simulink model "Modelo_Diferencial"  (R2019a)
settings: Solver=VariableStepAuto  StartTime=0.0  StopTime=500  RelTol=1e-3
model workspace (MAT data in the model file):
  P = [0.118997681558  0.340385726666  0.751267059306; 0.498364051982  0.58526775098  0.255095115459; 0.959743958516  0.223811939491  0.505957051665]
  xe = [0; 0; 0]
undefined symbols (not defined in the file or in its folder): sigbuilder_block
libraries: simulink x1
settings Model: OrderedModelArguments=off  Creator=Steven  LastModifiedBy=PC-88464
settings DataIOCC: ReturnWorkspaceOutputs=off
settings DebuggingCC: ArithmeticOperatorsInVariantConditions=warning
settings SFSimCC: SimUseLocalCustomCode=off
settings RTWCC: RTWUseLocalCustomCode=off
settings CodeAppCC: StateflowObjectComments=on

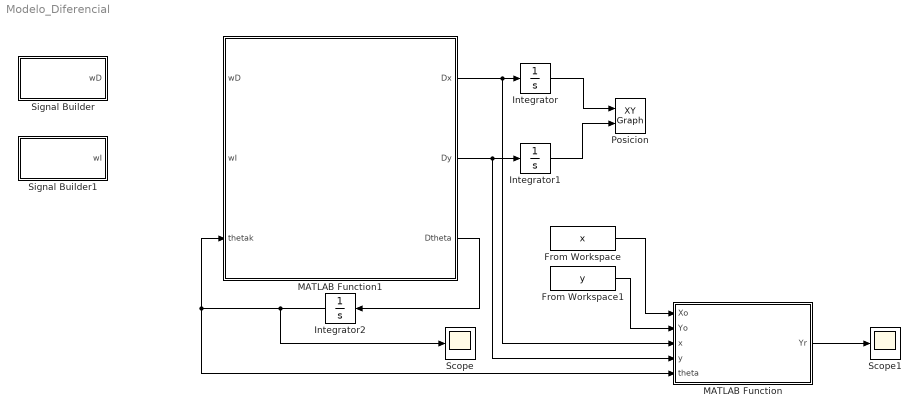
== system Modelo_Diferencial ==
  From Workspace : FromWorkspace  VariableName=x  SampleTime=0
  From Workspace1 : FromWorkspace  VariableName=y  SampleTime=0
  Integrator : Integrator
  Integrator1 : Integrator
  Integrator2 : Integrator
  MATLAB Function : MATLAB Function  TreatAsAtomicUnit=on
  MATLAB Function1 : MATLAB Function  TreatAsAtomicUnit=on  SystemSampleTime=0.5
  Posicion : simulink/Sinks/XY Graph  xmin=-100  xmax=100  ymin=-10  ymax=200  st=0.5
  Scope : Scope
  Scope1 : Scope
  Signal Builder : Subsystem  Tag=STV Subsys  LoadFcn=sigbuilder_block('load');  StartFcn=sigbuilder_block('start');  StopFcn=sigbuilder_block('stop');  ClipboardFcn=sigbuilder_block('clipboard');  mask(Sigbuilder block){tuvar=[0:10]}
      mask help: Simulink:masks:SigbuilderBlock_MD
      mask init:
      | if ~strcmp(get_param(bdroot(gcbh),'SimulationStatus'),'stopped') tuvar = sigbuilder_block('maskInit'); end
      settings: CopyFcn=sigbuilder_block('copy');  DeleteFcn=sigbuilder_block('delete');  ModelCloseFcn=sigbuilder_block('modelClose');  PreSaveFcn=sigbuilder_block('preSave');  PauseFcn=sigbuilder_block('pause');  ContinueFcn=sigbuilder_block('continue');  NameChangeFcn=sigbuilder_block('namechange');  OpenFcn=sigbuilder_block('open',[0.75 276.75 510.75 211.5 ]);  CloseFcn=sigbuilder_block('close');
      mask Display: plot(0, 0, 100, 100,[2, 2, 32, 32, 2], [68, 8, 8, 68, 68],[32, 2], [38, 38], [32, 19, 2],[53, 60, 44], [32, 17, 17, 2],[16, 16, 31, 31]);txt = getActiveGroup(gcbh);text(2, 100, txt,'verticalAlignment', 'top');
  Signal Builder1 : Subsystem  Tag=STV Subsys  LoadFcn=sigbuilder_block('load');  StartFcn=sigbuilder_block('start');  StopFcn=sigbuilder_block('stop');  ClipboardFcn=sigbuilder_block('clipboard');  mask(Sigbuilder block){tuvar=[0:10]}
      mask help: Simulink:masks:SigbuilderBlock_MD
      mask init:
      | if ~strcmp(get_param(bdroot(gcbh),'SimulationStatus'),'stopped') tuvar = sigbuilder_block('maskInit'); end
      settings: CopyFcn=sigbuilder_block('copy');  DeleteFcn=sigbuilder_block('delete');  ModelCloseFcn=sigbuilder_block('modelClose');  PreSaveFcn=sigbuilder_block('preSave');  PauseFcn=sigbuilder_block('pause');  ContinueFcn=sigbuilder_block('continue');  NameChangeFcn=sigbuilder_block('namechange');  OpenFcn=sigbuilder_block('open',[0.75 0.75 510.75 211.5 ]);  CloseFcn=sigbuilder_block('close');
      mask Display: plot(0, 0, 100, 100,[2, 2, 32, 32, 2], [68, 8, 8, 68, 68],[32, 2], [38, 38], [32, 19, 2],[53, 60, 44], [32, 17, 17, 2],[16, 16, 31, 31]);txt = getActiveGroup(gcbh);text(2, 100, txt,'verticalAlignment', 'top');
  wires:
  MATLAB Function1/3(Dtheta) -> Integrator2/1
  Integrator2/1 -> Scope/1, MATLAB Function/5(theta), MATLAB Function1/3(thetak)
  MATLAB Function1/1(Dx) -> MATLAB Function/3(x), Integrator/1
  MATLAB Function1/2(Dy) -> MATLAB Function/4(y), Integrator1/1
  Integrator/1 -> Posicion/1
  Integrator1/1 -> Posicion/2
  From Workspace/1 -> MATLAB Function/1(Xo)
  From Workspace1/1 -> MATLAB Function/2(Yo)
  MATLAB Function/1(Yr) -> Scope1/1

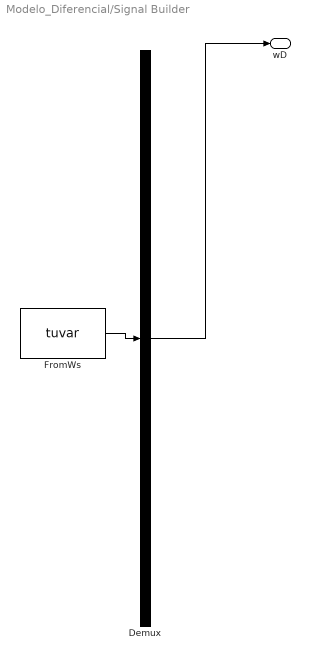
== system Modelo_Diferencial/Signal Builder ==
  Demux : Demux  Tag=STV Demux  Outputs=1
  FromWs : FromWorkspace  Tag=STV FromWs  VariableName=tuvar  SampleTime=0
      SigBuilderData=|
      | common.afterFinalStr = 'Extrapolate'
      | common.sampleTime = 0
      | dataSet.timeRange = [0 500]
      | dataSet.name = 'Group 1'
      | sbobj.Groups.Name = 'Group 1'
      | sbobj.Groups.Signals.Name = 'wD'
      | sbobj.Groups.Signals.XData = [0 11.2 11.2 24.5 24.5 33.8 33.8 500]
      | sbobj.Groups.Signals.YData = [9.9 9.9 8 8.00092555332 6 6 3 3]
      | sbobj.Groups.TimeRange = [0 500]
  wD : Outport  Tag=STV Outport
  wires:
  Demux/1 -> wD/1
  FromWs/1 -> Demux/1

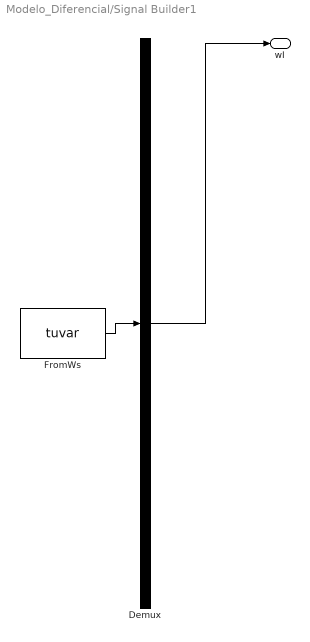
== system Modelo_Diferencial/Signal Builder1 ==
  Demux : Demux  Tag=STV Demux  Outputs=1
  FromWs : FromWorkspace  Tag=STV FromWs  VariableName=tuvar  SampleTime=0
      SigBuilderData=|
      | common.afterFinalStr = 'Extrapolate'
      | common.sampleTime = 0
      | dataSet.timeRange = [0 500]
      | dataSet.name = 'Group 1'
      | sbobj.Groups.Name = 'Group 1'
      | sbobj.Groups.Signals.Name = 'wI'
      | sbobj.Groups.Signals.XData = [0 500]
      | sbobj.Groups.Signals.YData = [5 5]
      | sbobj.Groups.TimeRange = [0 500]
  wI : Outport  Tag=STV Outport
  wires:
  Demux/1 -> wI/1
  FromWs/1 -> Demux/1

== matlab function Modelo_Diferencial/MATLAB Function1 ==
  data: wD input; wI input; Dx output; Dy output; thetak input; Dtheta output
function [Dx,Dy,Dtheta] = modelo(wD,wI,thetak)
Ts = 0.5;
r = 1.2;
b = 19.5;
B= [(r*(Ts*cos(thetak))/2) (r*(Ts*cos(thetak))/2);(r*(Ts*sin(thetak)/2)) (r*(Ts*sin(thetak)/2));(Ts*(r/b)) (Ts*(-r/b))];
u= [ wD; wI];

out =(B*u);
Dx=out(1);
Dy=out(2);
Dtheta=out(3);

== matlab function Modelo_Diferencial/MATLAB Function ==
  data: Xo input; Yr output; Yo input; x input; y input; theta input
function Yr = seguimiento(Xo,Yo,x,y,theta)
%hallamos parametro L correspondiente 
L = sqrt(((Xo-x).^2)+((Yo-y).^2));
Dx = (((Xo-x)*cos(theta))+((Yo-y)*sin(theta)));

r=(()/2*Dx)
%velocidad lineal de cada rueda
vI=v*(1-(b/2*r));
vD=v*(1+(b/2*r));

Yr = (2*Dx/L.^2);
